simulink model "np"  (R2024a)
settings: Solver=VariableStepAuto  StartTime=0.0  StopTime=4000  RelTol=1e-3
libraries: aerolibatmos2 x25, simulink x1
(part 1 of 3)
settings Model: Creator=NAILSK  LastModifiedBy=NAILSK

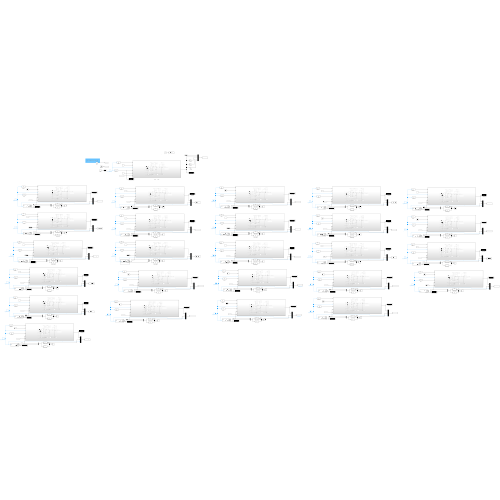
[thumbnail: Simulink's stored preview of the top-level diagram]
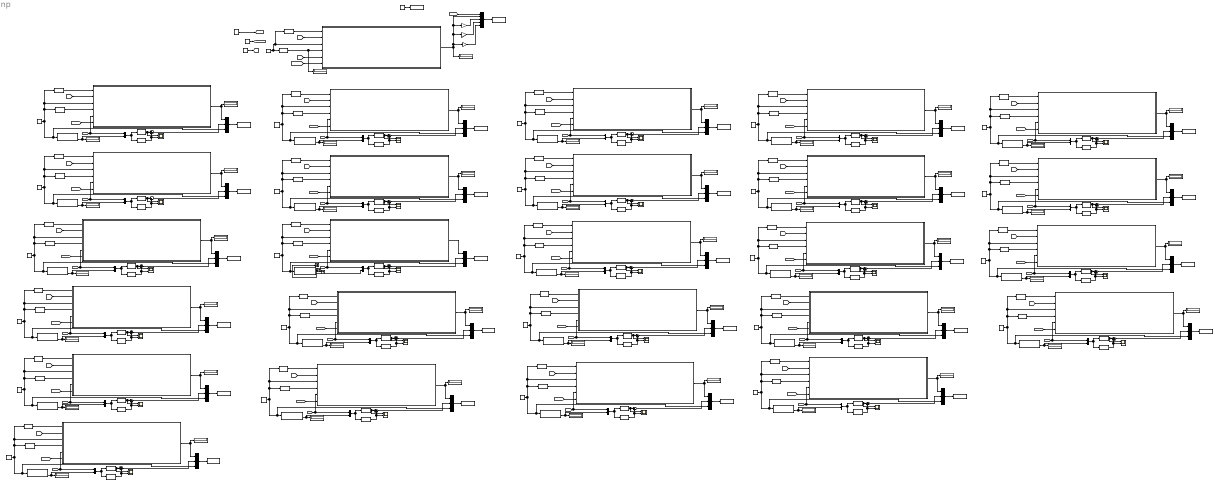
== system np ==
  note: stop time 2000 and slope .1 always works
  note: f=6.271
  note: e=.883
  50%SSL : Gain  Gain=.5
  65%SSL : Gain  Gain=0.65
  75%SSL : Gain  Gain=0.75
  COESA Atmosphere Model{,1..24} (25 alike) : aerolibatmos2/COESA Atmosphere Model  units=English (Velocity in ft/s)  spec=1976 COESA-extended U.S. Standard Atmosphere  model=Profile  profile_var=High temperature  profile_percent=1%  profile_alt=5 km (16404 ft)  envelope_var=High temperature  envelope_percent=1%  action=Warning
  Display{1..26} (26 alike) : Display
  Induced Drag{,1..24} (25 alike) : Fcn  Expr=2/(u[2]*pi*0.883)*(2250/36.1)^2*(1/u[1]^2)
  MAP{1..26} (26 alike) : Fcn  Expr=0.98*29.92*(1-u[1]/145442)^5.255876
  Mux{1..2,6,8..9,12,16,18..19,22,24..26,28,30,32,34,36,38,40..41,44,46,48,50} (25 alike) : Mux  Inputs=3
  Mux{3..4,7,10..11,13..15,17,20..21,23,27,29,31,33,35,37,39,42..43,45,47,49,51} (25 alike) : Mux  Inputs=2
  Mux5 : Mux  Inputs=5
  OAT{1..26} (26 alike) : Fcn  Expr=(519-0.00357*u[1])-459.67
  Parasite Drag{,1..24} (25 alike) : Fcn  Expr=0.5*u[2]*u[1]^2*6.271
  RPM : Constant  Value=2700
  Scope{,1..24} (25 alike) : Scope  NumInputPorts=2
  Subsystem : Subsystem
  Subsystem1 : Subsystem
  Subsystem10 : Subsystem
  Subsystem11 : Subsystem
  Subsystem12 : Subsystem
  Subsystem13 : Subsystem
  Subsystem14 : Subsystem
  Subsystem15 : Subsystem
  Subsystem16 : Subsystem
  Subsystem17 : Subsystem
  Subsystem18 : Subsystem
  Subsystem19 : Subsystem
  Subsystem2 : Subsystem
  Subsystem20 : Subsystem
  Subsystem21 : Subsystem
  Subsystem22 : Subsystem
  Subsystem23 : Subsystem
  Subsystem24 : Subsystem
  Subsystem25 : Subsystem
  Subsystem3 : Subsystem
  Subsystem4 : Subsystem
  Subsystem5 : Subsystem
  Subsystem6 : Subsystem
  Subsystem7 : Subsystem
  Subsystem8 : Subsystem
  Subsystem9 : Subsystem
  Sum{,1..24} (25 alike) : Sum  Inputs=|++
  Terminator : Terminator
  Terminator1 : Terminator
  Terminator2 : Terminator
  This is just to set my inherited sample time : Constant
  Thrust (lb){,1..23} (24 alike) : Display
  To Workspace : ToWorkspace  VariableName=sealevel  SampleTime=-1
  To Workspace1 : ToWorkspace  VariableName=One  SampleTime=-1
  To Workspace10 : ToWorkspace  VariableName=Ten  SampleTime=-1
  To Workspace11 : ToWorkspace  VariableName=Eleven  SampleTime=-1
  To Workspace12 : ToWorkspace  VariableName=Twelve  SampleTime=-1
  To Workspace13 : ToWorkspace  VariableName=Thirteen  SampleTime=-1
  To Workspace14 : ToWorkspace  VariableName=Fourteen  SampleTime=-1
  To Workspace15 : ToWorkspace  VariableName=Fifteen  SampleTime=-1
  To Workspace16 : ToWorkspace  VariableName=Sixteen  SampleTime=-1
  To Workspace17 : ToWorkspace  VariableName=Eighteen  SampleTime=-1
  To Workspace18 : ToWorkspace  VariableName=Seventeen  SampleTime=-1
  To Workspace19 : ToWorkspace  VariableName=Nineteen  SampleTime=-1
  To Workspace2 : ToWorkspace  VariableName=Two  SampleTime=-1
  To Workspace20 : ToWorkspace  VariableName=dummy  SampleTime=1
  To Workspace21 : ToWorkspace  VariableName=OneFive  SampleTime=-1
  To Workspace22 : ToWorkspace  VariableName=TwoFive  SampleTime=-1
  To Workspace23 : ToWorkspace  VariableName=TwelveFive  SampleTime=-1
  To Workspace24 : ToWorkspace  VariableName=NineFive  SampleTime=-1
  To Workspace25 : ToWorkspace  VariableName=ThirteenFive  SampleTime=-1
  To Workspace26 : ToWorkspace  VariableName=Zero  SampleTime=-1
  To Workspace3 : ToWorkspace  VariableName=Three  SampleTime=-1
  To Workspace4 : ToWorkspace  VariableName=Four  SampleTime=-1
  To Workspace5 : ToWorkspace  VariableName=Five  SampleTime=-1
  To Workspace6 : ToWorkspace  VariableName=Six  SampleTime=-1
  To Workspace7 : ToWorkspace  VariableName=Seven  SampleTime=-1
  To Workspace8 : ToWorkspace  VariableName=Eight  SampleTime=-1
  To Workspace9 : ToWorkspace  VariableName=Nine  SampleTime=-1
  Vtas : simulink/Sources/Ramp  slope=.05  start=0  InitialOutput=40
  diameter1 : Constant  Value=6.14
  hp (pressure alt) : Constant  Value=1000
  hp (pressure alt)1 : Constant  Value=0
  hp (pressure alt)10 : Constant  Value=10000
  hp (pressure alt)11 : Constant  Value=11000
  hp (pressure alt)12 : Constant  Value=12000
  hp (pressure alt)13 : Constant  Value=13000
  hp (pressure alt)14 : Constant  Value=14000
  hp (pressure alt)15 : Constant  Value=15000
  hp (pressure alt)16 : Constant  Value=16000
  hp (pressure alt)17 : Constant  Value=18000
  hp (pressure alt)18 : Constant  Value=17000
  hp (pressure alt)19 : Constant  Value=19000
  hp (pressure alt)2 : Constant  Value=2000
  hp (pressure alt)20 : Constant  Value=1500
  hp (pressure alt)21 : Constant  Value=2500
  hp (pressure alt)22 : Constant  Value=12500
  hp (pressure alt)23 : Constant  Value=9500
  hp (pressure alt)24 : Constant  Value=13500
  hp (pressure alt)25 : Constant  Value=0
  hp (pressure alt)3 : Constant  Value=3000
  hp (pressure alt)4 : Constant  Value=4000
  hp (pressure alt)5 : Constant  Value=5000
  hp (pressure alt)6 : Constant  Value=6000
  hp (pressure alt)7 : Constant  Value=7000
  hp (pressure alt)8 : Constant  Value=8000
  hp (pressure alt)9 : Constant  Value=9000
  wires:
  Mux4/1 -> Parasite Drag/1, Induced Drag/1
  COESA Atmosphere Model/4 -> Display3/1, Mux4/2
  Parasite Drag/1 -> Scope/1, Sum/1
  Induced Drag/1 -> Scope/2, Sum/2
  Mux5/1 -> To Workspace/1
  Sum/1 -> Mux1/2
  [Vtas] -> Mux4/1, Subsystem/5(In5)
  Subsystem/1(Out1) -> Mux1/1, Thrust (lb)/1
  hp (pressure alt)/1 -> OAT2/1, MAP2/1, Subsystem/3(In3), Mux1/3, COESA Atmosphere Model/1
  OAT2/1 -> Subsystem/4(In4)
  hp (pressure alt)1/1 -> MAP3/1, Subsystem1/3(In3), OAT1/1
  MAP3/1 -> Subsystem1/1(In1)
  OAT1/1 -> Display1/1, Subsystem1/4(In4)
  Subsystem1/1(Out1) -> 50%SSL/1, 65%SSL/1, Mux5/2, 75%SSL/1, Display2/1
  Vtas/1 -> [Vtas]
  [Vtas] -> Subsystem1/5(In5)
  [Vtas] -> Mux5/1
  75%SSL/1 -> Mux5/3
  65%SSL/1 -> Mux5/4
  50%SSL/1 -> Mux5/5
  Mux1/1 -> To Workspace1/1
  diameter1/1 -> [Diameter]
  [Diameter] -> Subsystem1/6(In6)
  [Diameter] -> Subsystem/6(In6)
  RPM/1 -> [RPM]
  [RPM] -> Subsystem1/2(In2)
  [RPM] -> Subsystem/2(In2)
  MAP2/1 -> Subsystem/1(In1)
  MAP1/1 -> Subsystem2/1(In1)
  [RPM] -> Subsystem2/2(In2)
  [Diameter] -> Subsystem2/6(In6)
  Mux2/1 -> To Workspace2/1
  OAT3/1 -> Subsystem2/4(In4)
  hp (pressure alt)2/1 -> COESA Atmosphere Model1/1, Mux2/3, Subsystem2/3(In3), MAP1/1, OAT3/1
  Subsystem2/1(Out1) -> Thrust (lb)1/1, Mux2/1
  [Vtas] -> Subsystem2/5(In5), Mux3/1
  Sum1/1 -> Mux2/2
  Induced Drag1/1 -> Sum1/2, Scope1/2
  Parasite Drag1/1 -> Sum1/1, Scope1/1
  COESA Atmosphere Model1/4 -> Mux3/2, Display4/1
  Mux3/1 -> Induced Drag1/1, Parasite Drag1/1
  Mux7/1 -> Parasite Drag2/1, Induced Drag2/1
  COESA Atmosphere Model2/4 -> Mux7/2
  Parasite Drag2/1 -> Scope2/1, Sum2/1
  Induced Drag2/1 -> Scope2/2, Sum2/2
  Sum2/1 -> Mux6/2
  [Vtas] -> Mux7/1, Subsystem3/5(In5)
  Subsystem3/1(Out1) -> Mux6/1
  hp (pressure alt)3/1 -> OAT4/1, MAP4/1, Subsystem3/3(In3), Mux6/3, COESA Atmosphere Model2/1
  OAT4/1 -> Subsystem3/4(In4)
  Mux6/1 -> To Workspace3/1
  [Diameter] -> Subsystem3/6(In6)
  [RPM] -> Subsystem3/2(In2)
  MAP4/1 -> Subsystem3/1(In1)
  MAP7/1 -> Subsystem6/1(In1)
  [RPM] -> Subsystem6/2(In2)
  [Diameter] -> Subsystem6/6(In6)
  Mux12/1 -> To Workspace6/1
  OAT7/1 -> Subsystem6/4(In4)
  hp (pressure alt)6/1 -> COESA Atmosphere Model5/1, Mux12/3, Subsystem6/3(In3), MAP7/1, OAT7/1
  Subsystem6/1(Out1) -> Thrust (lb)5/1, Mux12/1
  [Vtas] -> Subsystem6/5(In5), Mux13/1
  Sum5/1 -> Mux12/2
  Induced Drag5/1 -> Sum5/2, Scope5/2
  Parasite Drag5/1 -> Sum5/1, Scope5/1
  COESA Atmosphere Model5/4 -> Mux13/2, Display8/1
  Mux13/1 -> Induced Drag5/1, Parasite Drag5/1
  Mux10/1 -> Parasite Drag4/1, Induced Drag4/1
  COESA Atmosphere Model4/4 -> Display7/1, Mux10/2
  Parasite Drag4/1 -> Scope4/1, Sum4/1
  Induced Drag4/1 -> Scope4/2, Sum4/2
  Sum4/1 -> Mux9/2
  [Vtas] -> Mux10/1, Subsystem5/5(In5)
  Subsystem5/1(Out1) -> Mux9/1, Thrust (lb)4/1
  hp (pressure alt)5/1 -> OAT6/1, MAP5/1, Subsystem5/3(In3), Mux9/3, COESA Atmosphere Model4/1
  OAT6/1 -> Subsystem5/4(In4)
  Mux9/1 -> To Workspace5/1
  [Diameter] -> Subsystem5/6(In6)
  [RPM] -> Subsystem5/2(In2)
  MAP5/1 -> Subsystem5/1(In1)
  MAP6/1 -> Subsystem4/1(In1)
  [RPM] -> Subsystem4/2(In2)
  [Diameter] -> Subsystem4/6(In6)
  Mux8/1 -> To Workspace4/1
  OAT5/1 -> Subsystem4/4(In4)
  hp (pressure alt)4/1 -> COESA Atmosphere Model3/1, Mux8/3, Subsystem4/3(In3), MAP6/1, OAT5/1
  Subsystem4/1(Out1) -> Thrust (lb)3/1, Mux8/1
  [Vtas] -> Subsystem4/5(In5), Mux11/1
  Sum3/1 -> Mux8/2
  Induced Drag3/1 -> Sum3/2, Scope3/2
  Parasite Drag3/1 -> Sum3/1, Scope3/1
  COESA Atmosphere Model3/4 -> Mux11/2, Display6/1
  Mux11/1 -> Induced Drag3/1, Parasite Drag3/1
  Mux15/1 -> Parasite Drag6/1, Induced Drag6/1
  COESA Atmosphere Model6/4 -> Display9/1, Mux15/2
  Parasite Drag6/1 -> Scope6/1, Sum6/1
  Induced Drag6/1 -> Scope6/2, Sum6/2
  Sum6/1 -> Mux18/2
  [Vtas] -> Mux15/1, Subsystem7/5(In5)
  Subsystem7/1(Out1) -> Mux18/1, Thrust (lb)6/1
  hp (pressure alt)7/1 -> OAT8/1, MAP9/1, Subsystem7/3(In3), Mux18/3, COESA Atmosphere Model6/1
  OAT8/1 -> Subsystem7/4(In4)
  Mux18/1 -> To Workspace7/1
  [Diameter] -> Subsystem7/6(In6)
  [RPM] -> Subsystem7/2(In2)
  MAP9/1 -> Subsystem7/1(In1)
  MAP8/1 -> Subsystem8/1(In1)
  [RPM] -> Subsystem8/2(In2)
  [Diameter] -> Subsystem8/6(In6)
  Mux19/1 -> To Workspace8/1
  OAT9/1 -> Subsystem8/4(In4)
  hp (pressure alt)8/1 -> COESA Atmosphere Model7/1, Mux19/3, Subsystem8/3(In3), MAP8/1, OAT9/1
  Subsystem8/1(Out1) -> Thrust (lb)7/1, Mux19/1
  [Vtas] -> Subsystem8/5(In5), Mux14/1
  Sum7/1 -> Mux19/2
  Induced Drag7/1 -> Sum7/2, Scope7/2
  Parasite Drag7/1 -> Sum7/1, Scope7/1
  COESA Atmosphere Model7/4 -> Mux14/2, Display10/1
  Mux14/1 -> Induced Drag7/1, Parasite Drag7/1
  Mux17/1 -> Parasite Drag8/1, Induced Drag8/1
  COESA Atmosphere Model8/4 -> Display11/1, Mux17/2
  Parasite Drag8/1 -> Scope8/1, Sum8/1
  Induced Drag8/1 -> Scope8/2, Sum8/2
  Sum8/1 -> Mux16/2
  [Vtas] -> Mux17/1, Subsystem9/5(In5)
  Subsystem9/1(Out1) -> Mux16/1, Thrust (lb)8/1
  hp (pressure alt)9/1 -> OAT10/1, MAP10/1, Subsystem9/3(In3), Mux16/3, COESA Atmosphere Model8/1
  OAT10/1 -> Subsystem9/4(In4)
  Mux16/1 -> To Workspace9/1
  [Diameter] -> Subsystem9/6(In6)
  [RPM] -> Subsystem9/2(In2)
  MAP10/1 -> Subsystem9/1(In1)
  MAP11/1 -> Subsystem12/1(In1)
  [RPM] -> Subsystem12/2(In2)
  [Diameter] -> Subsystem12/6(In6)
  Mux22/1 -> To Workspace12/1
  OAT11/1 -> Subsystem12/4(In4)
  hp (pressure alt)12/1 -> COESA Atmosphere Model11/1, Mux22/3, Subsystem12/3(In3), MAP11/1, OAT11/1
  Subsystem12/1(Out1) -> Thrust (lb)11/1, Mux22/1
  [Vtas] -> Subsystem12/5(In5), Mux23/1
  Sum11/1 -> Mux22/2
  Induced Drag11/1 -> Sum11/2, Scope11/2
  Parasite Drag11/1 -> Sum11/1, Scope11/1
  COESA Atmosphere Model11/4 -> Mux23/2, Display13/1
  Mux23/1 -> Induced Drag11/1, Parasite Drag11/1
  Mux20/1 -> Parasite Drag10/1, Induced Drag10/1
  COESA Atmosphere Model10/4 -> Display12/1, Mux20/2
  Parasite Drag10/1 -> Scope10/1, Sum10/1
  Induced Drag10/1 -> Scope10/2, Sum10/2
  Sum10/1 -> Mux25/2
  [Vtas] -> Mux20/1, Subsystem11/5(In5)
  Subsystem11/1(Out1) -> Mux25/1, Thrust (lb)10/1
  hp (pressure alt)11/1 -> OAT13/1, MAP12/1, Subsystem11/3(In3), Mux25/3, COESA Atmosphere Model10/1
  OAT13/1 -> Subsystem11/4(In4)
  Mux25/1 -> To Workspace11/1
  [Diameter] -> Subsystem11/6(In6)
  [RPM] -> Subsystem11/2(In2)
  MAP12/1 -> Subsystem11/1(In1)
  MAP13/1 -> Subsystem10/1(In1)
  [RPM] -> Subsystem10/2(In2)
  [Diameter] -> Subsystem10/6(In6)
  Mux24/1 -> To Workspace10/1
  OAT12/1 -> Subsystem10/4(In4)
  hp (pressure alt)10/1 -> COESA Atmosphere Model9/1, Mux24/3, Subsystem10/3(In3), MAP13/1, OAT12/1
  Subsystem10/1(Out1) -> Thrust (lb)9/1, Mux24/1
  [Vtas] -> Subsystem10/5(In5), Mux21/1
  Sum9/1 -> Mux24/2
  Induced Drag9/1 -> Sum9/2, Scope9/2
  Parasite Drag9/1 -> Sum9/1, Scope9/1
  COESA Atmosphere Model9/4 -> Mux21/2, Display14/1
  Mux21/1 -> Induced Drag9/1, Parasite Drag9/1
  COESA Atmosphere Model2/3 -> Terminator/1
  COESA Atmosphere Model2/2 -> Terminator1/1
  COESA Atmosphere Model2/1 -> Terminator2/1
  [RPM] -> Subsystem13/2(In2)
  Induced Drag12/1 -> Sum12/2, Scope12/2
  [Vtas] -> Subsystem13/5(In5), Mux27/1
  COESA Atmosphere Model12/4 -> Mux27/2, Display5/1
  Parasite Drag12/1 -> Sum12/1, Scope12/1
  Mux27/1 -> Induced Drag12/1, Parasite Drag12/1
  Sum12/1 -> Mux26/2
  Mux26/1 -> To Workspace13/1
  MAP14/1 -> Subsystem13/1(In1)
  Subsystem13/1(Out1) -> Thrust (lb)2/1, Mux26/1
  [Diameter] -> Subsystem13/6(In6)
  hp (pressure alt)13/1 -> COESA Atmosphere Model12/1, Mux26/3, Subsystem13/3(In3), MAP14/1, OAT14/1
  OAT14/1 -> Subsystem13/4(In4)
  [RPM] -> Subsystem14/2(In2)
  Induced Drag13/1 -> Sum13/2, Scope13/2
  [Vtas] -> Subsystem14/5(In5), Mux29/1
  COESA Atmosphere Model13/4 -> Mux29/2, Display15/1
  Parasite Drag13/1 -> Sum13/1, Scope13/1
  Mux29/1 -> Induced Drag13/1, Parasite Drag13/1
  Sum13/1 -> Mux28/2
  Mux28/1 -> To Workspace14/1
  MAP15/1 -> Subsystem14/1(In1)
  Subsystem14/1(Out1) -> Thrust (lb)12/1, Mux28/1
  [Diameter] -> Subsystem14/6(In6)
  hp (pressure alt)14/1 -> COESA Atmosphere Model13/1, Mux28/3, Subsystem14/3(In3), MAP15/1, OAT15/1
  OAT15/1 -> Subsystem14/4(In4)
  [RPM] -> Subsystem15/2(In2)
  Induced Drag14/1 -> Sum14/2, Scope14/2
  [Vtas] -> Subsystem15/5(In5), Mux31/1
  COESA Atmosphere Model14/4 -> Mux31/2, Display16/1
  Parasite Drag14/1 -> Sum14/1, Scope14/1
  Mux31/1 -> Induced Drag14/1, Parasite Drag14/1
  Sum14/1 -> Mux30/2
  Mux30/1 -> To Workspace15/1
  MAP16/1 -> Subsystem15/1(In1)
  Subsystem15/1(Out1) -> Thrust (lb)13/1, Mux30/1
  [Diameter] -> Subsystem15/6(In6)
  hp (pressure alt)15/1 -> COESA Atmosphere Model14/1, Mux30/3, Subsystem15/3(In3), MAP16/1, OAT16/1
  OAT16/1 -> Subsystem15/4(In4)
  [Vtas] -> Subsystem16/5(In5), Mux33/1
  [RPM] -> Subsystem16/2(In2)
  Induced Drag15/1 -> Sum15/2, Scope15/2
  OAT17/1 -> Subsystem16/4(In4)
  [Diameter] -> Subsystem16/6(In6)
  hp (pressure alt)16/1 -> COESA Atmosphere Model15/1, Mux32/3, Subsystem16/3(In3), MAP17/1, OAT17/1
  Subsystem16/1(Out1) -> Thrust (lb)14/1, Mux32/1
  Parasite Drag15/1 -> Sum15/1, Scope15/1
  Mux32/1 -> To Workspace16/1
  Mux33/1 -> Induced Drag15/1, Parasite Drag15/1
  COESA Atmosphere Model15/4 -> Mux33/2, Display17/1
  MAP17/1 -> Subsystem16/1(In1)
  Sum15/1 -> Mux32/2
  Sum16/1 -> Mux34/2
  MAP18/1 -> Subsystem17/1(In1)
  COESA Atmosphere Model16/4 -> Display18/1, Mux35/2
  Mux35/1 -> Parasite Drag16/1, Induced Drag16/1
  Mux34/1 -> To Workspace17/1
  Parasite Drag16/1 -> Scope16/1, Sum16/1
  Subsystem17/1(Out1) -> Mux34/1, Thrust (lb)15/1
  hp (pressure alt)17/1 -> OAT18/1, MAP18/1, Subsystem17/3(In3), Mux34/3, COESA Atmosphere Model16/1
  [Diameter] -> Subsystem17/6(In6)
  OAT18/1 -> Subsystem17/4(In4)
  Induced Drag16/1 -> Scope16/2, Sum16/2
  [RPM] -> Subsystem17/2(In2)
  [Vtas] -> Mux35/1, Subsystem17/5(In5)
  [Vtas] -> Subsystem18/5(In5), Mux37/1
  [RPM] -> Subsystem18/2(In2)
  Induced Drag17/1 -> Sum17/2, Scope17/2
  OAT19/1 -> Subsystem18/4(In4)
  [Diameter] -> Subsystem18/6(In6)
  hp (pressure alt)18/1 -> COESA Atmosphere Model17/1, Mux36/3, Subsystem18/3(In3), MAP19/1, OAT19/1
  Subsystem18/1(Out1) -> Thrust (lb)16/1, Mux36/1
  Parasite Drag17/1 -> Sum17/1, Scope17/1
  Mux36/1 -> To Workspace18/1
  Mux37/1 -> Induced Drag17/1, Parasite Drag17/1
  COESA Atmosphere Model17/4 -> Mux37/2, Display19/1
  MAP19/1 -> Subsystem18/1(In1)
  Sum17/1 -> Mux36/2
  [Vtas] -> Subsystem19/5(In5), Mux39/1
  [RPM] -> Subsystem19/2(In2)
  Induced Drag18/1 -> Sum18/2, Scope18/2
  OAT20/1 -> Subsystem19/4(In4)
  [Diameter] -> Subsystem19/6(In6)
  hp (pressure alt)19/1 -> COESA Atmosphere Model18/1, Mux38/3, Subsystem19/3(In3), MAP20/1, OAT20/1
  Subsystem19/1(Out1) -> Thrust (lb)17/1, Mux38/1
  Parasite Drag18/1 -> Sum18/1, Scope18/1
  Mux38/1 -> To Workspace19/1
  Mux39/1 -> Induced Drag18/1, Parasite Drag18/1
  COESA Atmosphere Model18/4 -> Mux39/2, Display20/1
  MAP20/1 -> Subsystem19/1(In1)
  Sum18/1 -> Mux38/2
  This is just to set my inherited sample time/1 -> To Workspace20/1
  Mux42/1 -> Parasite Drag20/1, Induced Drag20/1
  COESA Atmosphere Model20/4 -> Display22/1, Mux42/2
  Parasite Drag20/1 -> Scope20/1, Sum20/1
  Induced Drag20/1 -> Scope20/2, Sum20/2
  Sum20/1 -> Mux41/2
  [Vtas] -> Mux42/1, Subsystem21/5(In5)
  Subsystem21/1(Out1) -> Mux41/1, Thrust (lb)19/1
  hp (pressure alt)21/1 -> OAT22/1, MAP21/1, Subsystem21/3(In3), Mux41/3, COESA Atmosphere Model20/1
  OAT22/1 -> Subsystem21/4(In4)
  Mux41/1 -> To Workspace22/1
  [Diameter] -> Subsystem21/6(In6)
  [RPM] -> Subsystem21/2(In2)
  MAP21/1 -> Subsystem21/1(In1)
  MAP22/1 -> Subsystem20/1(In1)
  [RPM] -> Subsystem20/2(In2)
  [Diameter] -> Subsystem20/6(In6)
  Mux40/1 -> To Workspace21/1
  OAT21/1 -> Subsystem20/4(In4)
  hp (pressure alt)20/1 -> COESA Atmosphere Model19/1, Mux40/3, Subsystem20/3(In3), MAP22/1, OAT21/1
  Subsystem20/1(Out1) -> Thrust (lb)18/1, Mux40/1
  [Vtas] -> Subsystem20/5(In5), Mux43/1
  Sum19/1 -> Mux40/2
  Induced Drag19/1 -> Sum19/2, Scope19/2
  Parasite Drag19/1 -> Sum19/1, Scope19/1
  COESA Atmosphere Model19/4 -> Mux43/2, Display21/1
  Mux43/1 -> Induced Drag19/1, Parasite Drag19/1
  MAP23/1 -> Subsystem22/1(In1)
  [RPM] -> Subsystem22/2(In2)
  [Diameter] -> Subsystem22/6(In6)
  Mux44/1 -> To Workspace23/1
  OAT23/1 -> Subsystem22/4(In4)
  hp (pressure alt)22/1 -> COESA Atmosphere Model21/1, Mux44/3, Subsystem22/3(In3), MAP23/1, OAT23/1
  Subsystem22/1(Out1) -> Thrust (lb)20/1, Mux44/1
  [Vtas] -> Subsystem22/5(In5), Mux45/1
  Sum21/1 -> Mux44/2
  Induced Drag21/1 -> Sum21/2, Scope21/2
  Parasite Drag21/1 -> Sum21/1, Scope21/1
  COESA Atmosphere Model21/4 -> Mux45/2, Display23/1
  Mux45/1 -> Induced Drag21/1, Parasite Drag21/1
  Mux47/1 -> Parasite Drag22/1, Induced Drag22/1
  COESA Atmosphere Model22/4 -> Display24/1, Mux47/2
  Parasite Drag22/1 -> Scope22/1, Sum22/1
  Induced Drag22/1 -> Scope22/2, Sum22/2
  Sum22/1 -> Mux46/2
  [Vtas] -> Mux47/1, Subsystem23/5(In5)
  Subsystem23/1(Out1) -> Mux46/1, Thrust (lb)21/1
  hp (pressure alt)23/1 -> OAT24/1, MAP24/1, Subsystem23/3(In3), Mux46/3, COESA Atmosphere Model22/1
  OAT24/1 -> Subsystem23/4(In4)
  Mux46/1 -> To Workspace24/1
  [Diameter] -> Subsystem23/6(In6)
  [RPM] -> Subsystem23/2(In2)
  MAP24/1 -> Subsystem23/1(In1)
  MAP25/1 -> Subsystem24/1(In1)
  [RPM] -> Subsystem24/2(In2)
  [Diameter] -> Subsystem24/6(In6)
  Mux48/1 -> To Workspace25/1
  OAT25/1 -> Subsystem24/4(In4)
  hp (pressure alt)24/1 -> COESA Atmosphere Model23/1, Mux48/3, Subsystem24/3(In3), MAP25/1, OAT25/1
  Subsystem24/1(Out1) -> Thrust (lb)22/1, Mux48/1
  [Vtas] -> Subsystem24/5(In5), Mux49/1
  Sum23/1 -> Mux48/2
  Induced Drag23/1 -> Sum23/2, Scope23/2
  Parasite Drag23/1 -> Sum23/1, Scope23/1
  COESA Atmosphere Model23/4 -> Mux49/2, Display25/1
  Mux49/1 -> Induced Drag23/1, Parasite Drag23/1
  Mux51/1 -> Parasite Drag24/1, Induced Drag24/1
  COESA Atmosphere Model24/4 -> Display26/1, Mux51/2
  Parasite Drag24/1 -> Scope24/1, Sum24/1
  Induced Drag24/1 -> Scope24/2, Sum24/2
  Sum24/1 -> Mux50/2
  [Vtas] -> Mux51/1, Subsystem25/5(In5)
  Subsystem25/1(Out1) -> Mux50/1, Thrust (lb)23/1
  hp (pressure alt)25/1 -> OAT26/1, MAP26/1, Subsystem25/3(In3), Mux50/3, COESA Atmosphere Model24/1
  OAT26/1 -> Subsystem25/4(In4)
  Mux50/1 -> To Workspace26/1
  [Diameter] -> Subsystem25/6(In6)
  [RPM] -> Subsystem25/2(In2)
  MAP26/1 -> Subsystem25/1(In1)

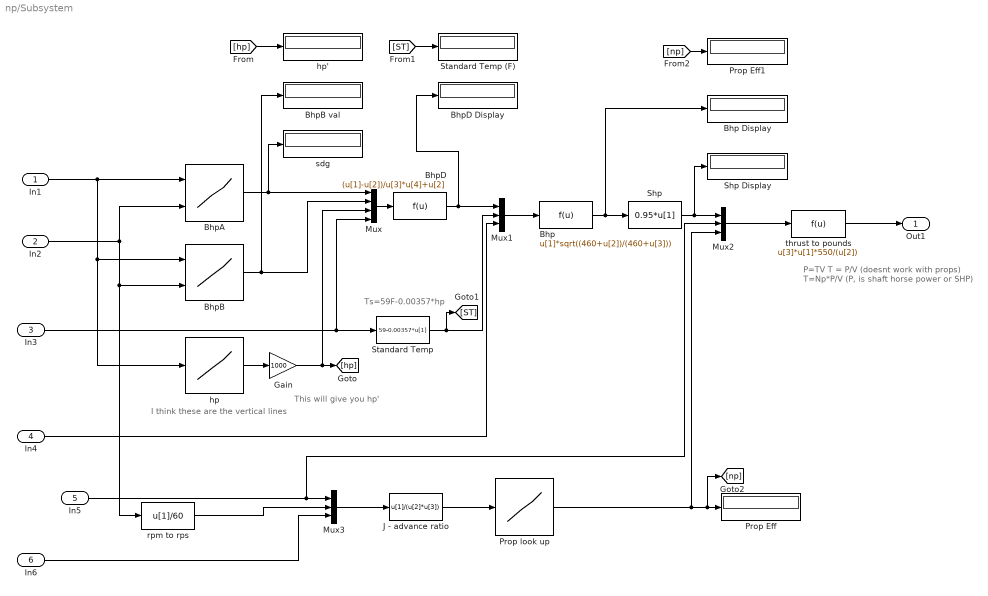
== system np/Subsystem ==
  note: I think these are the vertical lines
  note: Ts=59F-0.00357*hp
  note: P=TV
      |
      | T = P/V (doesnt work with props)
      | T=Np*P/V (P, is shaft horse power or SHP)
  note: This will give you hp'
  In1 : Inport
  In2 : Inport  Port=2
  In3 : Inport  Port=3
  In4 : Inport  Port=4
  In5 : Inport  Port=5
  In6 : Inport  Port=6
  Bhp : Fcn  Expr=u[1]*sqrt((460+u[2])/(460+u[3]))
  Bhp Display : Display
  BhpA : Lookup_n-D  BreakpointsForDimension1=[12;14;16;18;20;22;24;26;28]  BreakpointsForDimension2=[2000 2200 2400 2600 2700]  Table=[55 65 68 70 71;69 77 82 84 87;79 87 94 97 100;88 98 105 111 115;98 108 116 123 126;108 119 127 135 140;119 129 138 147 153;127 139 150 160 164;138 149 161 172 177]  InternalRulePriority=Speed  RndMeth=Simplest
      settings: InputPortMap=u0,u1
  BhpB : Lookup_n-D  BreakpointsForDimension1=[17 18 19 20 21 22 23 24 25 26 27 28 29]  BreakpointsForDimension2=[2000 2200 2400 2600 2700]  Table=[60 68 71 81 82;65 74 80 98 90;73 81 86 95 98;80 87 94 103 106;85 95 102 111 116;93 103 110 120 123;100 110 118 126 133;106 115 125 135 141;116 124 135 144 150;120 131 143 152 158;125 137 148 159 165;135 145 157 167 173;142 153 165 176 183]  InternalRulePriority=Speed  RndMeth=Simplest
      settings: InputPortMap=u0,u1
  BhpB val : Display
  BhpD : Fcn  Expr=(u[1]-u[2])/u[3]*u[4]+u[2]
  BhpD Display : Display
  Gain : Gain  Gain=1000
  J - advance ratio : Fcn  Expr=u[1]/(u[2]*u[3])
  Mux : Mux
  Mux1 : Mux  Inputs=3
  Mux2 : Mux  Inputs=3
  Mux3 : Mux  Inputs=3
  Prop Eff : Display
  Prop Eff1 : Display
  Prop look up : Lookup_n-D  NumberOfTableDimensions=1  BreakpointsForDimension1=[0;0.048012249;0.060807878;0.079983697;0.105563205;0.133281193;0.157430152;0.178753263;0.199368443;0.215001671;0.227800237;0.245557257;0.273971426;0.300949171;0.327207235;0.352754431;0.371192944;0.390339388;0.409494645;0.433608354;0.457002383;0.472603298;0.491041811;0.509471512;0.534281402;0.552003172;0.576810125;0.598782418;0.619332973;0.645549913;0.671763915;0.690895672;0.717103799;0.745432781;0.760302266;0.778708467;0.799946391;0.819051711;0.845926644;0.867848999;0.888343743;0.903180915;0.92013013;0.934250559;0.947645432;0.961736487;0.970184657;0.980736057;0.986337817;0.992650444;0.994753675]  Table=[0;0.109900628;0.134509301;0.163123953;0.206809061;0.257361734;0.294163365;0.333794761;0.373442069;0.400753217;0.42674495;0.454008364;0.499012887;0.534367813;0.564206411;0.592677861;0.607477825;0.622261878;0.641195111;0.661400024;0.676088609;0.688186099;0.702986063;0.713636848;0.72829361;0.738960306;0.752234009;0.764188297;0.773408288;0.783884048;0.792976749;0.800845502;0.807172083;0.81206787;0.813116793;0.812703099;0.812225759;0.807646975;0.794594806;0.783037077;0.765978931;0.751814195;0.732069486;0.713771482;0.68719103;0.655062427;0.632742534;0.600693488;0.571521941;0.543717542;0.53398839]  InternalRulePriority=Speed  RndMeth=Simplest
  Shp : Fcn  Expr=0.95*u[1]
  Shp Display : Display
  Standard Temp : Fcn  Expr=59-0.00357*u[1]
  Standard Temp (F) : Display
  hp : Lookup_n-D  NumberOfTableDimensions=1  BreakpointsForDimension1=[12, 14, 16, 18, 20, 22, 24, 26, 28]  Table=[22.5, 19.3, 15.8, 12.8, 10.3, 7.8, 5.5, 3.25, 1.4]  InternalRulePriority=Speed  RndMeth=Simplest
  "hp' " : Display
  rpm to rps : Fcn  Expr=u[1]/60
  sdg : Display
  thrust to pounds : Fcn  Expr=u[3]*u[1]*550/(u[2])
  Out1 : Outport
  wires:
  hp/1 -> Gain/1
  Gain/1 -> [hp], Mux/3
  [ST] -> Standard Temp (F)/1
  Mux3/1 -> J - advance ratio/1
  [hp] -> "hp' "/1
  rpm to rps/1 -> Mux3/2
  Mux/1 -> BhpD/1
  Prop look up/1 -> [np], Prop Eff/1, Mux2/3
  J - advance ratio/1 -> Prop look up/1
  [np] -> Prop Eff1/1
  Shp/1 -> Shp Display/1, Mux2/1
  In1/1 -> hp/1, BhpB/1, BhpA/1
  In2/1 -> BhpA/2, BhpB/2, rpm to rps/1
  Mux1/1 -> Bhp/1
  BhpB/1 -> BhpB val/1, Mux/2
  Standard Temp/1 -> [ST], Mux1/2
  In3/1 -> Mux/4, Standard Temp/1
  thrust to pounds/1 -> Out1/1
  Bhp/1 -> Bhp Display/1, Shp/1
  In5/1 -> Mux2/2, Mux3/1
  Mux2/1 -> thrust to pounds/1
  BhpD/1 -> BhpD Display/1, Mux1/1
  BhpA/1 -> sdg/1, Mux/1
  In4/1 -> Mux1/3
  In6/1 -> Mux3/3

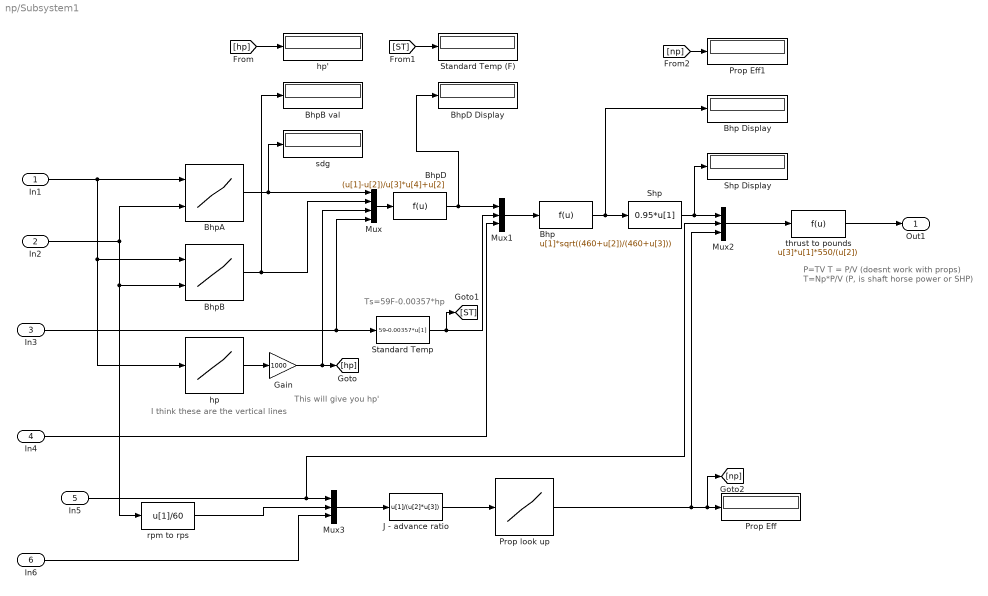
== system np/Subsystem1 ==
  note: This will give you hp'
  note: P=TV
      |
      | T = P/V (doesnt work with props)
      | T=Np*P/V (P, is shaft horse power or SHP)
  note: Ts=59F-0.00357*hp
  note: I think these are the vertical lines
  In1 : Inport
  In2 : Inport  Port=2
  In3 : Inport  Port=3
  In4 : Inport  Port=4
  In5 : Inport  Port=5
  In6 : Inport  Port=6
  Bhp : Fcn  Expr=u[1]*sqrt((460+u[2])/(460+u[3]))
  Bhp Display : Display
  BhpA : Lookup_n-D  BreakpointsForDimension1=[12;14;16;18;20;22;24;26;28]  BreakpointsForDimension2=[2000 2200 2400 2600 2700]  Table=[55 65 68 70 71;69 77 82 84 87;79 87 94 97 100;88 98 105 111 115;98 108 116 123 126;108 119 127 135 140;119 129 138 147 153;127 139 150 160 164;138 149 161 172 177]  InternalRulePriority=Speed  RndMeth=Simplest
      settings: InputPortMap=u0,u1
  BhpB : Lookup_n-D  BreakpointsForDimension1=[17 18 19 20 21 22 23 24 25 26 27 28 29]  BreakpointsForDimension2=[2000 2200 2400 2600 2700]  Table=[60 68 71 81 82;65 74 80 98 90;73 81 86 95 98;80 87 94 103 106;85 95 102 111 116;93 103 110 120 123;100 110 118 126 133;106 115 125 135 141;116 124 135 144 150;120 131 143 152 158;125 137 148 159 165;135 145 157 167 173;142 153 165 176 183]  InternalRulePriority=Speed  RndMeth=Simplest
      settings: InputPortMap=u0,u1
  BhpB val : Display
  BhpD : Fcn  Expr=(u[1]-u[2])/u[3]*u[4]+u[2]
  BhpD Display : Display
  Gain : Gain  Gain=1000
  J - advance ratio : Fcn  Expr=u[1]/(u[2]*u[3])
  Mux : Mux
  Mux1 : Mux  Inputs=3
  Mux2 : Mux  Inputs=3
  Mux3 : Mux  Inputs=3
  Prop Eff : Display
  Prop Eff1 : Display
  Prop look up : Lookup_n-D  NumberOfTableDimensions=1  BreakpointsForDimension1=[0;0.048012249;0.060807878;0.079983697;0.105563205;0.133281193;0.157430152;0.178753263;0.199368443;0.215001671;0.227800237;0.245557257;0.273971426;0.300949171;0.327207235;0.352754431;0.371192944;0.390339388;0.409494645;0.433608354;0.457002383;0.472603298;0.491041811;0.509471512;0.534281402;0.552003172;0.576810125;0.598782418;0.619332973;0.645549913;0.671763915;0.690895672;0.717103799;0.745432781;0.760302266;0.778708467;0.799946391;0.819051711;0.845926644;0.867848999;0.888343743;0.903180915;0.92013013;0.934250559;0.947645432;0.961736487;0.970184657;0.980736057;0.986337817;0.992650444;0.994753675]  Table=[0;0.109900628;0.134509301;0.163123953;0.206809061;0.257361734;0.294163365;0.333794761;0.373442069;0.400753217;0.42674495;0.454008364;0.499012887;0.534367813;0.564206411;0.592677861;0.607477825;0.622261878;0.641195111;0.661400024;0.676088609;0.688186099;0.702986063;0.713636848;0.72829361;0.738960306;0.752234009;0.764188297;0.773408288;0.783884048;0.792976749;0.800845502;0.807172083;0.81206787;0.813116793;0.812703099;0.812225759;0.807646975;0.794594806;0.783037077;0.765978931;0.751814195;0.732069486;0.713771482;0.68719103;0.655062427;0.632742534;0.600693488;0.571521941;0.543717542;0.53398839]  InternalRulePriority=Speed  RndMeth=Simplest
  Shp : Fcn  Expr=0.95*u[1]
  Shp Display : Display
  Standard Temp : Fcn  Expr=59-0.00357*u[1]
  Standard Temp (F) : Display
  hp : Lookup_n-D  NumberOfTableDimensions=1  BreakpointsForDimension1=[12, 14, 16, 18, 20, 22, 24, 26, 28]  Table=[22.5, 19.3, 15.8, 12.8, 10.3, 7.8, 5.5, 3.25, 1.4]  InternalRulePriority=Speed  RndMeth=Simplest
  "hp' " : Display
  rpm to rps : Fcn  Expr=u[1]/60
  sdg : Display
  thrust to pounds : Fcn  Expr=u[3]*u[1]*550/(u[2])
  Out1 : Outport
  wires:
  In6/1 -> Mux3/3
  In4/1 -> Mux1/3
  BhpA/1 -> Mux/1, sdg/1
  BhpD/1 -> Mux1/1, BhpD Display/1
  Mux2/1 -> thrust to pounds/1
  In5/1 -> Mux3/1, Mux2/2
  Bhp/1 -> Shp/1, Bhp Display/1
  thrust to pounds/1 -> Out1/1
  In3/1 -> Standard Temp/1, Mux/4
  Standard Temp/1 -> Mux1/2, [ST]
  BhpB/1 -> Mux/2, BhpB val/1
  Mux1/1 -> Bhp/1
  In2/1 -> rpm to rps/1, BhpB/2, BhpA/2
  In1/1 -> BhpA/1, BhpB/1, hp/1
  Shp/1 -> Mux2/1, Shp Display/1
  [np] -> Prop Eff1/1
  J - advance ratio/1 -> Prop look up/1
  Prop look up/1 -> Mux2/3, Prop Eff/1, [np]
  Mux/1 -> BhpD/1
  rpm to rps/1 -> Mux3/2
  [hp] -> "hp' "/1
  Mux3/1 -> J - advance ratio/1
  [ST] -> Standard Temp (F)/1
  Gain/1 -> Mux/3, [hp]
  hp/1 -> Gain/1

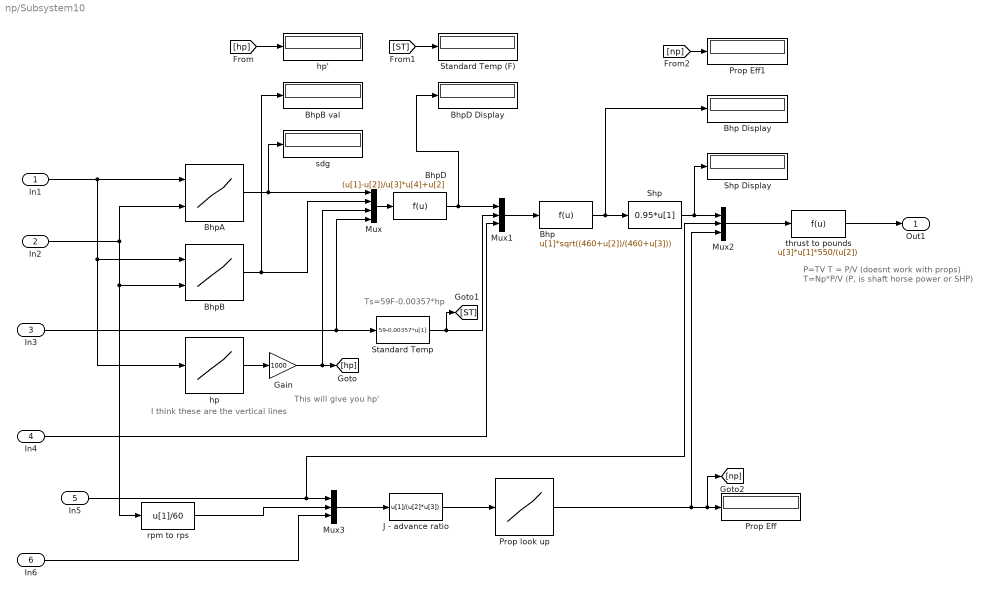
== system np/Subsystem10 ==
  note: This will give you hp'
  note: P=TV
      |
      | T = P/V (doesnt work with props)
      | T=Np*P/V (P, is shaft horse power or SHP)
  note: Ts=59F-0.00357*hp
  note: I think these are the vertical lines
  In1 : Inport
  In2 : Inport  Port=2
  In3 : Inport  Port=3
  In4 : Inport  Port=4
  In5 : Inport  Port=5
  In6 : Inport  Port=6
  Bhp : Fcn  Expr=u[1]*sqrt((460+u[2])/(460+u[3]))
  Bhp Display : Display
  BhpA : Lookup_n-D  BreakpointsForDimension1=[12;14;16;18;20;22;24;26;28]  BreakpointsForDimension2=[2000 2200 2400 2600 2700]  Table=[55 65 68 70 71;69 77 82 84 87;79 87 94 97 100;88 98 105 111 115;98 108 116 123 126;108 119 127 135 140;119 129 138 147 153;127 139 150 160 164;138 149 161 172 177]  InternalRulePriority=Speed  RndMeth=Simplest
      settings: InputPortMap=u0,u1
  BhpB : Lookup_n-D  BreakpointsForDimension1=[17 18 19 20 21 22 23 24 25 26 27 28 29]  BreakpointsForDimension2=[2000 2200 2400 2600 2700]  Table=[60 68 71 81 82;65 74 80 98 90;73 81 86 95 98;80 87 94 103 106;85 95 102 111 116;93 103 110 120 123;100 110 118 126 133;106 115 125 135 141;116 124 135 144 150;120 131 143 152 158;125 137 148 159 165;135 145 157 167 173;142 153 165 176 183]  InternalRulePriority=Speed  RndMeth=Simplest
      settings: InputPortMap=u0,u1
  BhpB val : Display
  BhpD : Fcn  Expr=(u[1]-u[2])/u[3]*u[4]+u[2]
  BhpD Display : Display
  Gain : Gain  Gain=1000
  J - advance ratio : Fcn  Expr=u[1]/(u[2]*u[3])
  Mux : Mux
  Mux1 : Mux  Inputs=3
  Mux2 : Mux  Inputs=3
  Mux3 : Mux  Inputs=3
  Prop Eff : Display
  Prop Eff1 : Display
  Prop look up : Lookup_n-D  NumberOfTableDimensions=1  BreakpointsForDimension1=[0;0.048012249;0.060807878;0.079983697;0.105563205;0.133281193;0.157430152;0.178753263;0.199368443;0.215001671;0.227800237;0.245557257;0.273971426;0.300949171;0.327207235;0.352754431;0.371192944;0.390339388;0.409494645;0.433608354;0.457002383;0.472603298;0.491041811;0.509471512;0.534281402;0.552003172;0.576810125;0.598782418;0.619332973;0.645549913;0.671763915;0.690895672;0.717103799;0.745432781;0.760302266;0.778708467;0.799946391;0.819051711;0.845926644;0.867848999;0.888343743;0.903180915;0.92013013;0.934250559;0.947645432;0.961736487;0.970184657;0.980736057;0.986337817;0.992650444;0.994753675]  Table=[0;0.109900628;0.134509301;0.163123953;0.206809061;0.257361734;0.294163365;0.333794761;0.373442069;0.400753217;0.42674495;0.454008364;0.499012887;0.534367813;0.564206411;0.592677861;0.607477825;0.622261878;0.641195111;0.661400024;0.676088609;0.688186099;0.702986063;0.713636848;0.72829361;0.738960306;0.752234009;0.764188297;0.773408288;0.783884048;0.792976749;0.800845502;0.807172083;0.81206787;0.813116793;0.812703099;0.812225759;0.807646975;0.794594806;0.783037077;0.765978931;0.751814195;0.732069486;0.713771482;0.68719103;0.655062427;0.632742534;0.600693488;0.571521941;0.543717542;0.53398839]  InternalRulePriority=Speed  RndMeth=Simplest
  Shp : Fcn  Expr=0.95*u[1]
  Shp Display : Display
  Standard Temp : Fcn  Expr=59-0.00357*u[1]
  Standard Temp (F) : Display
  hp : Lookup_n-D  NumberOfTableDimensions=1  BreakpointsForDimension1=[12, 14, 16, 18, 20, 22, 24, 26, 28]  Table=[22.5, 19.3, 15.8, 12.8, 10.3, 7.8, 5.5, 3.25, 1.4]  InternalRulePriority=Speed  RndMeth=Simplest
  "hp' " : Display
  rpm to rps : Fcn  Expr=u[1]/60
  sdg : Display
  thrust to pounds : Fcn  Expr=u[3]*u[1]*550/(u[2])
  Out1 : Outport
  wires:
  In6/1 -> Mux3/3
  In4/1 -> Mux1/3
  BhpA/1 -> Mux/1, sdg/1
  BhpD/1 -> Mux1/1, BhpD Display/1
  Mux2/1 -> thrust to pounds/1
  In5/1 -> Mux3/1, Mux2/2
  Bhp/1 -> Shp/1, Bhp Display/1
  thrust to pounds/1 -> Out1/1
  In3/1 -> Standard Temp/1, Mux/4
  Standard Temp/1 -> Mux1/2, [ST]
  BhpB/1 -> Mux/2, BhpB val/1
  Mux1/1 -> Bhp/1
  In2/1 -> rpm to rps/1, BhpB/2, BhpA/2
  In1/1 -> BhpA/1, BhpB/1, hp/1
  Shp/1 -> Mux2/1, Shp Display/1
  [np] -> Prop Eff1/1
  J - advance ratio/1 -> Prop look up/1
  Prop look up/1 -> Mux2/3, Prop Eff/1, [np]
  Mux/1 -> BhpD/1
  rpm to rps/1 -> Mux3/2
  [hp] -> "hp' "/1
  Mux3/1 -> J - advance ratio/1
  [ST] -> Standard Temp (F)/1
  Gain/1 -> Mux/3, [hp]
  hp/1 -> Gain/1

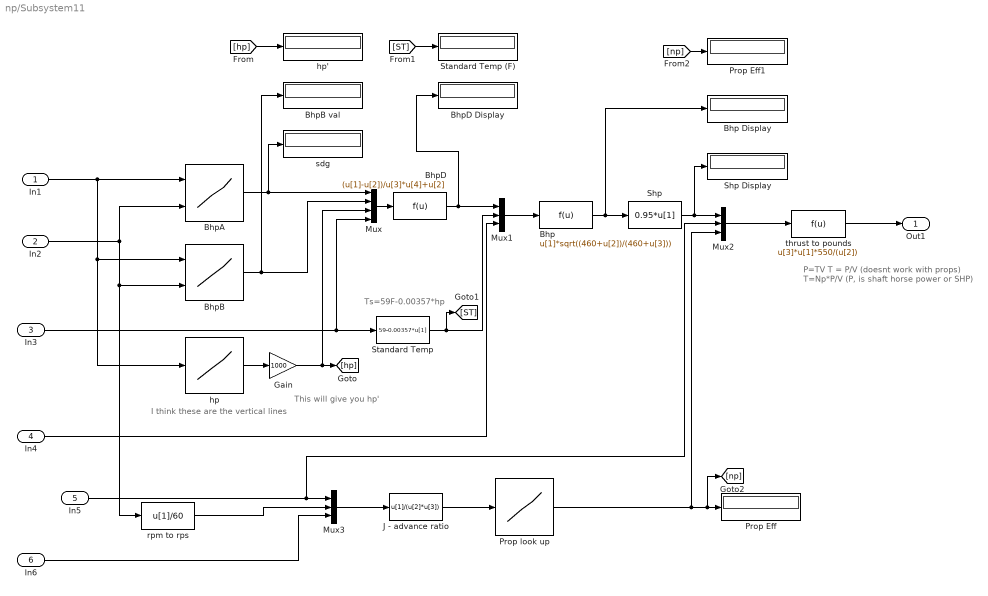
== system np/Subsystem11 ==
  note: I think these are the vertical lines
  note: Ts=59F-0.00357*hp
  note: P=TV
      |
      | T = P/V (doesnt work with props)
      | T=Np*P/V (P, is shaft horse power or SHP)
  note: This will give you hp'
  In1 : Inport
  In2 : Inport  Port=2
  In3 : Inport  Port=3
  In4 : Inport  Port=4
  In5 : Inport  Port=5
  In6 : Inport  Port=6
  Bhp : Fcn  Expr=u[1]*sqrt((460+u[2])/(460+u[3]))
  Bhp Display : Display
  BhpA : Lookup_n-D  BreakpointsForDimension1=[12;14;16;18;20;22;24;26;28]  BreakpointsForDimension2=[2000 2200 2400 2600 2700]  Table=[55 65 68 70 71;69 77 82 84 87;79 87 94 97 100;88 98 105 111 115;98 108 116 123 126;108 119 127 135 140;119 129 138 147 153;127 139 150 160 164;138 149 161 172 177]  InternalRulePriority=Speed  RndMeth=Simplest
      settings: InputPortMap=u0,u1
  BhpB : Lookup_n-D  BreakpointsForDimension1=[17 18 19 20 21 22 23 24 25 26 27 28 29]  BreakpointsForDimension2=[2000 2200 2400 2600 2700]  Table=[60 68 71 81 82;65 74 80 98 90;73 81 86 95 98;80 87 94 103 106;85 95 102 111 116;93 103 110 120 123;100 110 118 126 133;106 115 125 135 141;116 124 135 144 150;120 131 143 152 158;125 137 148 159 165;135 145 157 167 173;142 153 165 176 183]  InternalRulePriority=Speed  RndMeth=Simplest
      settings: InputPortMap=u0,u1
  BhpB val : Display
  BhpD : Fcn  Expr=(u[1]-u[2])/u[3]*u[4]+u[2]
  BhpD Display : Display
  Gain : Gain  Gain=1000
  J - advance ratio : Fcn  Expr=u[1]/(u[2]*u[3])
  Mux : Mux
  Mux1 : Mux  Inputs=3
  Mux2 : Mux  Inputs=3
  Mux3 : Mux  Inputs=3
  Prop Eff : Display
  Prop Eff1 : Display
  Prop look up : Lookup_n-D  NumberOfTableDimensions=1  BreakpointsForDimension1=[0;0.048012249;0.060807878;0.079983697;0.105563205;0.133281193;0.157430152;0.178753263;0.199368443;0.215001671;0.227800237;0.245557257;0.273971426;0.300949171;0.327207235;0.352754431;0.371192944;0.390339388;0.409494645;0.433608354;0.457002383;0.472603298;0.491041811;0.509471512;0.534281402;0.552003172;0.576810125;0.598782418;0.619332973;0.645549913;0.671763915;0.690895672;0.717103799;0.745432781;0.760302266;0.778708467;0.799946391;0.819051711;0.845926644;0.867848999;0.888343743;0.903180915;0.92013013;0.934250559;0.947645432;0.961736487;0.970184657;0.980736057;0.986337817;0.992650444;0.994753675]  Table=[0;0.109900628;0.134509301;0.163123953;0.206809061;0.257361734;0.294163365;0.333794761;0.373442069;0.400753217;0.42674495;0.454008364;0.499012887;0.534367813;0.564206411;0.592677861;0.607477825;0.622261878;0.641195111;0.661400024;0.676088609;0.688186099;0.702986063;0.713636848;0.72829361;0.738960306;0.752234009;0.764188297;0.773408288;0.783884048;0.792976749;0.800845502;0.807172083;0.81206787;0.813116793;0.812703099;0.812225759;0.807646975;0.794594806;0.783037077;0.765978931;0.751814195;0.732069486;0.713771482;0.68719103;0.655062427;0.632742534;0.600693488;0.571521941;0.543717542;0.53398839]  InternalRulePriority=Speed  RndMeth=Simplest
  Shp : Fcn  Expr=0.95*u[1]
  Shp Display : Display
  Standard Temp : Fcn  Expr=59-0.00357*u[1]
  Standard Temp (F) : Display
  hp : Lookup_n-D  NumberOfTableDimensions=1  BreakpointsForDimension1=[12, 14, 16, 18, 20, 22, 24, 26, 28]  Table=[22.5, 19.3, 15.8, 12.8, 10.3, 7.8, 5.5, 3.25, 1.4]  InternalRulePriority=Speed  RndMeth=Simplest
  "hp' " : Display
  rpm to rps : Fcn  Expr=u[1]/60
  sdg : Display
  thrust to pounds : Fcn  Expr=u[3]*u[1]*550/(u[2])
  Out1 : Outport
  wires:
  hp/1 -> Gain/1
  Gain/1 -> [hp], Mux/3
  [ST] -> Standard Temp (F)/1
  Mux3/1 -> J - advance ratio/1
  [hp] -> "hp' "/1
  rpm to rps/1 -> Mux3/2
  Mux/1 -> BhpD/1
  Prop look up/1 -> [np], Prop Eff/1, Mux2/3
  J - advance ratio/1 -> Prop look up/1
  [np] -> Prop Eff1/1
  Shp/1 -> Shp Display/1, Mux2/1
  In1/1 -> hp/1, BhpB/1, BhpA/1
  In2/1 -> BhpA/2, BhpB/2, rpm to rps/1
  Mux1/1 -> Bhp/1
  BhpB/1 -> BhpB val/1, Mux/2
  Standard Temp/1 -> [ST], Mux1/2
  In3/1 -> Mux/4, Standard Temp/1
  thrust to pounds/1 -> Out1/1
  Bhp/1 -> Bhp Display/1, Shp/1
  In5/1 -> Mux2/2, Mux3/1
  Mux2/1 -> thrust to pounds/1
  BhpD/1 -> BhpD Display/1, Mux1/1
  BhpA/1 -> sdg/1, Mux/1
  In4/1 -> Mux1/3
  In6/1 -> Mux3/3

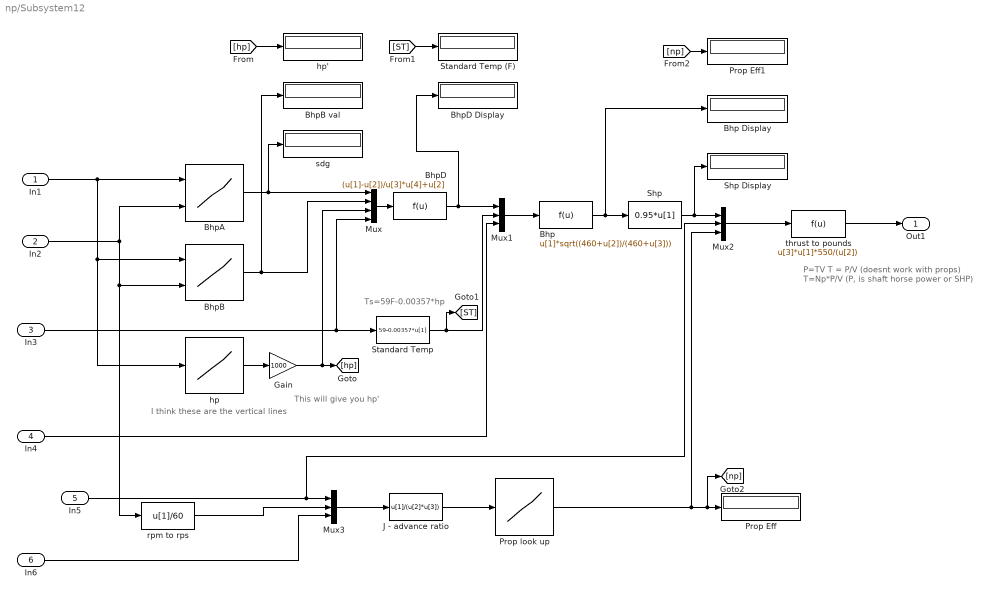
== system np/Subsystem12 ==
  note: This will give you hp'
  note: P=TV
      |
      | T = P/V (doesnt work with props)
      | T=Np*P/V (P, is shaft horse power or SHP)
  note: Ts=59F-0.00357*hp
  note: I think these are the vertical lines
  In1 : Inport
  In2 : Inport  Port=2
  In3 : Inport  Port=3
  In4 : Inport  Port=4
  In5 : Inport  Port=5
  In6 : Inport  Port=6
  Bhp : Fcn  Expr=u[1]*sqrt((460+u[2])/(460+u[3]))
  Bhp Display : Display
  BhpA : Lookup_n-D  BreakpointsForDimension1=[12;14;16;18;20;22;24;26;28]  BreakpointsForDimension2=[2000 2200 2400 2600 2700]  Table=[55 65 68 70 71;69 77 82 84 87;79 87 94 97 100;88 98 105 111 115;98 108 116 123 126;108 119 127 135 140;119 129 138 147 153;127 139 150 160 164;138 149 161 172 177]  InternalRulePriority=Speed  RndMeth=Simplest
      settings: InputPortMap=u0,u1
  BhpB : Lookup_n-D  BreakpointsForDimension1=[17 18 19 20 21 22 23 24 25 26 27 28 29]  BreakpointsForDimension2=[2000 2200 2400 2600 2700]  Table=[60 68 71 81 82;65 74 80 98 90;73 81 86 95 98;80 87 94 103 106;85 95 102 111 116;93 103 110 120 123;100 110 118 126 133;106 115 125 135 141;116 124 135 144 150;120 131 143 152 158;125 137 148 159 165;135 145 157 167 173;142 153 165 176 183]  InternalRulePriority=Speed  RndMeth=Simplest
      settings: InputPortMap=u0,u1
  BhpB val : Display
  BhpD : Fcn  Expr=(u[1]-u[2])/u[3]*u[4]+u[2]
  BhpD Display : Display
  Gain : Gain  Gain=1000
  J - advance ratio : Fcn  Expr=u[1]/(u[2]*u[3])
  Mux : Mux
  Mux1 : Mux  Inputs=3
  Mux2 : Mux  Inputs=3
  Mux3 : Mux  Inputs=3
  Prop Eff : Display
  Prop Eff1 : Display
  Prop look up : Lookup_n-D  NumberOfTableDimensions=1  BreakpointsForDimension1=[0;0.048012249;0.060807878;0.079983697;0.105563205;0.133281193;0.157430152;0.178753263;0.199368443;0.215001671;0.227800237;0.245557257;0.273971426;0.300949171;0.327207235;0.352754431;0.371192944;0.390339388;0.409494645;0.433608354;0.457002383;0.472603298;0.491041811;0.509471512;0.534281402;0.552003172;0.576810125;0.598782418;0.619332973;0.645549913;0.671763915;0.690895672;0.717103799;0.745432781;0.760302266;0.778708467;0.799946391;0.819051711;0.845926644;0.867848999;0.888343743;0.903180915;0.92013013;0.934250559;0.947645432;0.961736487;0.970184657;0.980736057;0.986337817;0.992650444;0.994753675]  Table=[0;0.109900628;0.134509301;0.163123953;0.206809061;0.257361734;0.294163365;0.333794761;0.373442069;0.400753217;0.42674495;0.454008364;0.499012887;0.534367813;0.564206411;0.592677861;0.607477825;0.622261878;0.641195111;0.661400024;0.676088609;0.688186099;0.702986063;0.713636848;0.72829361;0.738960306;0.752234009;0.764188297;0.773408288;0.783884048;0.792976749;0.800845502;0.807172083;0.81206787;0.813116793;0.812703099;0.812225759;0.807646975;0.794594806;0.783037077;0.765978931;0.751814195;0.732069486;0.713771482;0.68719103;0.655062427;0.632742534;0.600693488;0.571521941;0.543717542;0.53398839]  InternalRulePriority=Speed  RndMeth=Simplest
  Shp : Fcn  Expr=0.95*u[1]
  Shp Display : Display
  Standard Temp : Fcn  Expr=59-0.00357*u[1]
  Standard Temp (F) : Display
  hp : Lookup_n-D  NumberOfTableDimensions=1  BreakpointsForDimension1=[12, 14, 16, 18, 20, 22, 24, 26, 28]  Table=[22.5, 19.3, 15.8, 12.8, 10.3, 7.8, 5.5, 3.25, 1.4]  InternalRulePriority=Speed  RndMeth=Simplest
  "hp' " : Display
  rpm to rps : Fcn  Expr=u[1]/60
  sdg : Display
  thrust to pounds : Fcn  Expr=u[3]*u[1]*550/(u[2])
  Out1 : Outport
  wires:
  In6/1 -> Mux3/3
  In4/1 -> Mux1/3
  BhpA/1 -> Mux/1, sdg/1
  BhpD/1 -> Mux1/1, BhpD Display/1
  Mux2/1 -> thrust to pounds/1
  In5/1 -> Mux3/1, Mux2/2
  Bhp/1 -> Shp/1, Bhp Display/1
  thrust to pounds/1 -> Out1/1
  In3/1 -> Standard Temp/1, Mux/4
  Standard Temp/1 -> Mux1/2, [ST]
  BhpB/1 -> Mux/2, BhpB val/1
  Mux1/1 -> Bhp/1
  In2/1 -> rpm to rps/1, BhpB/2, BhpA/2
  In1/1 -> BhpA/1, BhpB/1, hp/1
  Shp/1 -> Mux2/1, Shp Display/1
  [np] -> Prop Eff1/1
  J - advance ratio/1 -> Prop look up/1
  Prop look up/1 -> Mux2/3, Prop Eff/1, [np]
  Mux/1 -> BhpD/1
  rpm to rps/1 -> Mux3/2
  [hp] -> "hp' "/1
  Mux3/1 -> J - advance ratio/1
  [ST] -> Standard Temp (F)/1
  Gain/1 -> Mux/3, [hp]
  hp/1 -> Gain/1

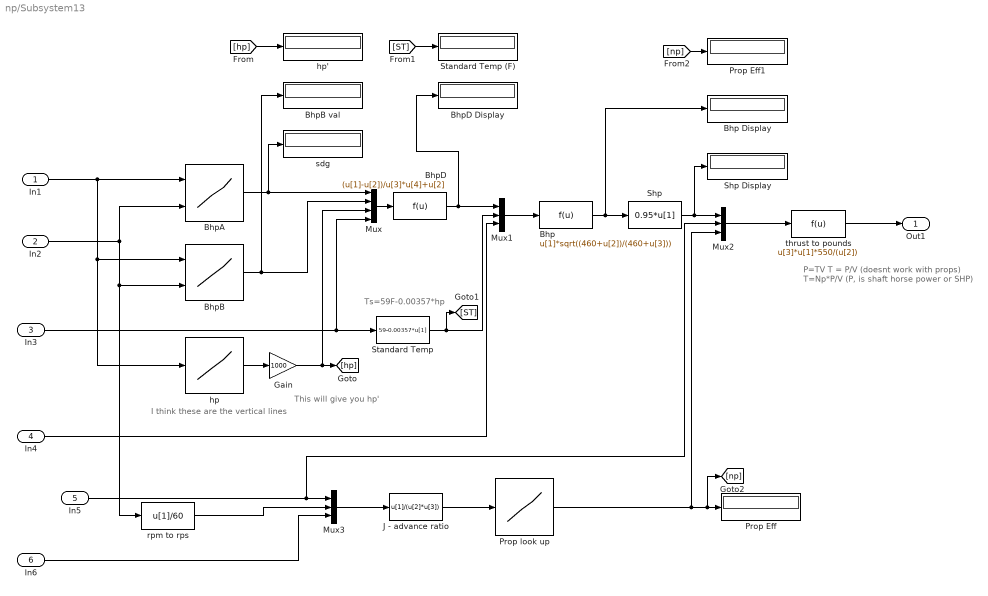
== system np/Subsystem13 ==
  note: This will give you hp'
  note: P=TV
      |
      | T = P/V (doesnt work with props)
      | T=Np*P/V (P, is shaft horse power or SHP)
  note: Ts=59F-0.00357*hp
  note: I think these are the vertical lines
  In1 : Inport
  In2 : Inport  Port=2
  In3 : Inport  Port=3
  In4 : Inport  Port=4
  In5 : Inport  Port=5
  In6 : Inport  Port=6
  Bhp : Fcn  Expr=u[1]*sqrt((460+u[2])/(460+u[3]))
  Bhp Display : Display
  BhpA : Lookup_n-D  BreakpointsForDimension1=[12;14;16;18;20;22;24;26;28]  BreakpointsForDimension2=[2000 2200 2400 2600 2700]  Table=[55 65 68 70 71;69 77 82 84 87;79 87 94 97 100;88 98 105 111 115;98 108 116 123 126;108 119 127 135 140;119 129 138 147 153;127 139 150 160 164;138 149 161 172 177]  InternalRulePriority=Speed  RndMeth=Simplest
      settings: InputPortMap=u0,u1
  BhpB : Lookup_n-D  BreakpointsForDimension1=[17 18 19 20 21 22 23 24 25 26 27 28 29]  BreakpointsForDimension2=[2000 2200 2400 2600 2700]  Table=[60 68 71 81 82;65 74 80 98 90;73 81 86 95 98;80 87 94 103 106;85 95 102 111 116;93 103 110 120 123;100 110 118 126 133;106 115 125 135 141;116 124 135 144 150;120 131 143 152 158;125 137 148 159 165;135 145 157 167 173;142 153 165 176 183]  InternalRulePriority=Speed  RndMeth=Simplest
      settings: InputPortMap=u0,u1
  BhpB val : Display
  BhpD : Fcn  Expr=(u[1]-u[2])/u[3]*u[4]+u[2]
  BhpD Display : Display
  Gain : Gain  Gain=1000
  J - advance ratio : Fcn  Expr=u[1]/(u[2]*u[3])
  Mux : Mux
  Mux1 : Mux  Inputs=3
  Mux2 : Mux  Inputs=3
  Mux3 : Mux  Inputs=3
  Prop Eff : Display
  Prop Eff1 : Display
  Prop look up : Lookup_n-D  NumberOfTableDimensions=1  BreakpointsForDimension1=[0;0.048012249;0.060807878;0.079983697;0.105563205;0.133281193;0.157430152;0.178753263;0.199368443;0.215001671;0.227800237;0.245557257;0.273971426;0.300949171;0.327207235;0.352754431;0.371192944;0.390339388;0.409494645;0.433608354;0.457002383;0.472603298;0.491041811;0.509471512;0.534281402;0.552003172;0.576810125;0.598782418;0.619332973;0.645549913;0.671763915;0.690895672;0.717103799;0.745432781;0.760302266;0.778708467;0.799946391;0.819051711;0.845926644;0.867848999;0.888343743;0.903180915;0.92013013;0.934250559;0.947645432;0.961736487;0.970184657;0.980736057;0.986337817;0.992650444;0.994753675]  Table=[0;0.109900628;0.134509301;0.163123953;0.206809061;0.257361734;0.294163365;0.333794761;0.373442069;0.400753217;0.42674495;0.454008364;0.499012887;0.534367813;0.564206411;0.592677861;0.607477825;0.622261878;0.641195111;0.661400024;0.676088609;0.688186099;0.702986063;0.713636848;0.72829361;0.738960306;0.752234009;0.764188297;0.773408288;0.783884048;0.792976749;0.800845502;0.807172083;0.81206787;0.813116793;0.812703099;0.812225759;0.807646975;0.794594806;0.783037077;0.765978931;0.751814195;0.732069486;0.713771482;0.68719103;0.655062427;0.632742534;0.600693488;0.571521941;0.543717542;0.53398839]  InternalRulePriority=Speed  RndMeth=Simplest
  Shp : Fcn  Expr=0.95*u[1]
  Shp Display : Display
  Standard Temp : Fcn  Expr=59-0.00357*u[1]
  Standard Temp (F) : Display
  hp : Lookup_n-D  NumberOfTableDimensions=1  BreakpointsForDimension1=[12, 14, 16, 18, 20, 22, 24, 26, 28]  Table=[22.5, 19.3, 15.8, 12.8, 10.3, 7.8, 5.5, 3.25, 1.4]  InternalRulePriority=Speed  RndMeth=Simplest
  "hp' " : Display
  rpm to rps : Fcn  Expr=u[1]/60
  sdg : Display
  thrust to pounds : Fcn  Expr=u[3]*u[1]*550/(u[2])
  Out1 : Outport
  wires:
  In6/1 -> Mux3/3
  In4/1 -> Mux1/3
  BhpA/1 -> Mux/1, sdg/1
  BhpD/1 -> Mux1/1, BhpD Display/1
  Mux2/1 -> thrust to pounds/1
  In5/1 -> Mux3/1, Mux2/2
  Bhp/1 -> Shp/1, Bhp Display/1
  thrust to pounds/1 -> Out1/1
  In3/1 -> Standard Temp/1, Mux/4
  Standard Temp/1 -> Mux1/2, [ST]
  BhpB/1 -> Mux/2, BhpB val/1
  Mux1/1 -> Bhp/1
  In2/1 -> rpm to rps/1, BhpB/2, BhpA/2
  In1/1 -> BhpA/1, BhpB/1, hp/1
  Shp/1 -> Mux2/1, Shp Display/1
  [np] -> Prop Eff1/1
  J - advance ratio/1 -> Prop look up/1
  Prop look up/1 -> Mux2/3, Prop Eff/1, [np]
  Mux/1 -> BhpD/1
  rpm to rps/1 -> Mux3/2
  [hp] -> "hp' "/1
  Mux3/1 -> J - advance ratio/1
  [ST] -> Standard Temp (F)/1
  Gain/1 -> Mux/3, [hp]
  hp/1 -> Gain/1

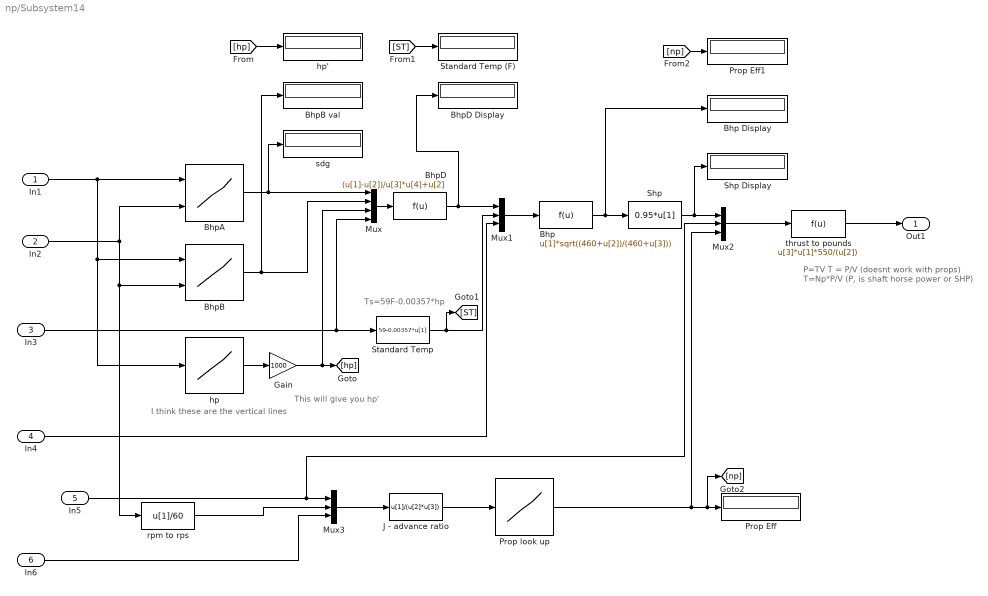
== system np/Subsystem14 ==
  note: This will give you hp'
  note: P=TV
      |
      | T = P/V (doesnt work with props)
      | T=Np*P/V (P, is shaft horse power or SHP)
  note: Ts=59F-0.00357*hp
  note: I think these are the vertical lines
  In1 : Inport
  In2 : Inport  Port=2
  In3 : Inport  Port=3
  In4 : Inport  Port=4
  In5 : Inport  Port=5
  In6 : Inport  Port=6
  Bhp : Fcn  Expr=u[1]*sqrt((460+u[2])/(460+u[3]))
  Bhp Display : Display
  BhpA : Lookup_n-D  BreakpointsForDimension1=[12;14;16;18;20;22;24;26;28]  BreakpointsForDimension2=[2000 2200 2400 2600 2700]  Table=[55 65 68 70 71;69 77 82 84 87;79 87 94 97 100;88 98 105 111 115;98 108 116 123 126;108 119 127 135 140;119 129 138 147 153;127 139 150 160 164;138 149 161 172 177]  InternalRulePriority=Speed  RndMeth=Simplest
      settings: InputPortMap=u0,u1
  BhpB : Lookup_n-D  BreakpointsForDimension1=[17 18 19 20 21 22 23 24 25 26 27 28 29]  BreakpointsForDimension2=[2000 2200 2400 2600 2700]  Table=[60 68 71 81 82;65 74 80 98 90;73 81 86 95 98;80 87 94 103 106;85 95 102 111 116;93 103 110 120 123;100 110 118 126 133;106 115 125 135 141;116 124 135 144 150;120 131 143 152 158;125 137 148 159 165;135 145 157 167 173;142 153 165 176 183]  InternalRulePriority=Speed  RndMeth=Simplest
      settings: InputPortMap=u0,u1
  BhpB val : Display
  BhpD : Fcn  Expr=(u[1]-u[2])/u[3]*u[4]+u[2]
  BhpD Display : Display
  Gain : Gain  Gain=1000
  J - advance ratio : Fcn  Expr=u[1]/(u[2]*u[3])
  Mux : Mux
  Mux1 : Mux  Inputs=3
  Mux2 : Mux  Inputs=3
  Mux3 : Mux  Inputs=3
  Prop Eff : Display
  Prop Eff1 : Display
  Prop look up : Lookup_n-D  NumberOfTableDimensions=1  BreakpointsForDimension1=[0;0.048012249;0.060807878;0.079983697;0.105563205;0.133281193;0.157430152;0.178753263;0.199368443;0.215001671;0.227800237;0.245557257;0.273971426;0.300949171;0.327207235;0.352754431;0.371192944;0.390339388;0.409494645;0.433608354;0.457002383;0.472603298;0.491041811;0.509471512;0.534281402;0.552003172;0.576810125;0.598782418;0.619332973;0.645549913;0.671763915;0.690895672;0.717103799;0.745432781;0.760302266;0.778708467;0.799946391;0.819051711;0.845926644;0.867848999;0.888343743;0.903180915;0.92013013;0.934250559;0.947645432;0.961736487;0.970184657;0.980736057;0.986337817;0.992650444;0.994753675]  Table=[0;0.109900628;0.134509301;0.163123953;0.206809061;0.257361734;0.294163365;0.333794761;0.373442069;0.400753217;0.42674495;0.454008364;0.499012887;0.534367813;0.564206411;0.592677861;0.607477825;0.622261878;0.641195111;0.661400024;0.676088609;0.688186099;0.702986063;0.713636848;0.72829361;0.738960306;0.752234009;0.764188297;0.773408288;0.783884048;0.792976749;0.800845502;0.807172083;0.81206787;0.813116793;0.812703099;0.812225759;0.807646975;0.794594806;0.783037077;0.765978931;0.751814195;0.732069486;0.713771482;0.68719103;0.655062427;0.632742534;0.600693488;0.571521941;0.543717542;0.53398839]  InternalRulePriority=Speed  RndMeth=Simplest
  Shp : Fcn  Expr=0.95*u[1]
  Shp Display : Display
  Standard Temp : Fcn  Expr=59-0.00357*u[1]
  Standard Temp (F) : Display
  hp : Lookup_n-D  NumberOfTableDimensions=1  BreakpointsForDimension1=[12, 14, 16, 18, 20, 22, 24, 26, 28]  Table=[22.5, 19.3, 15.8, 12.8, 10.3, 7.8, 5.5, 3.25, 1.4]  InternalRulePriority=Speed  RndMeth=Simplest
  "hp' " : Display
  rpm to rps : Fcn  Expr=u[1]/60
  sdg : Display
  thrust to pounds : Fcn  Expr=u[3]*u[1]*550/(u[2])
  Out1 : Outport
  wires:
  In6/1 -> Mux3/3
  In4/1 -> Mux1/3
  BhpA/1 -> Mux/1, sdg/1
  BhpD/1 -> Mux1/1, BhpD Display/1
  Mux2/1 -> thrust to pounds/1
  In5/1 -> Mux3/1, Mux2/2
  Bhp/1 -> Shp/1, Bhp Display/1
  thrust to pounds/1 -> Out1/1
  In3/1 -> Standard Temp/1, Mux/4
  Standard Temp/1 -> Mux1/2, [ST]
  BhpB/1 -> Mux/2, BhpB val/1
  Mux1/1 -> Bhp/1
  In2/1 -> rpm to rps/1, BhpB/2, BhpA/2
  In1/1 -> BhpA/1, BhpB/1, hp/1
  Shp/1 -> Mux2/1, Shp Display/1
  [np] -> Prop Eff1/1
  J - advance ratio/1 -> Prop look up/1
  Prop look up/1 -> Mux2/3, Prop Eff/1, [np]
  Mux/1 -> BhpD/1
  rpm to rps/1 -> Mux3/2
  [hp] -> "hp' "/1
  Mux3/1 -> J - advance ratio/1
  [ST] -> Standard Temp (F)/1
  Gain/1 -> Mux/3, [hp]
  hp/1 -> Gain/1
